simulink library "SKYWARD_LIB_2020b"  (R2020b)
settings: Solver=VariableStepAuto  StartTime=0.0  StopTime=10.0  RelTol=1e-3
undefined symbols (not defined in the file): A_d, CD, h0, I, m, q0, rho
libraries: $bdroot x2
settings Model: Creator=alem1  LastModifiedBy=aless

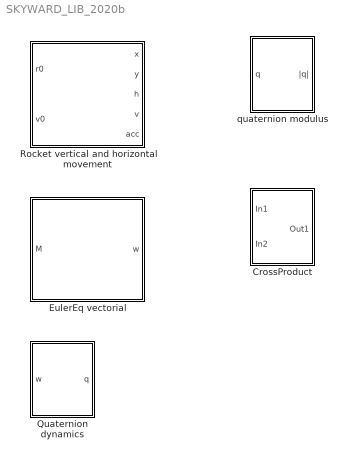
== system SKYWARD_LIB_2020b ==
  CrossProduct : Subsystem
  EulerEq vectorial : Subsystem
  Quaternion dynamics : Subsystem
  Rocket vertical and horizontal movement : Subsystem
  quaternion modulus : Subsystem

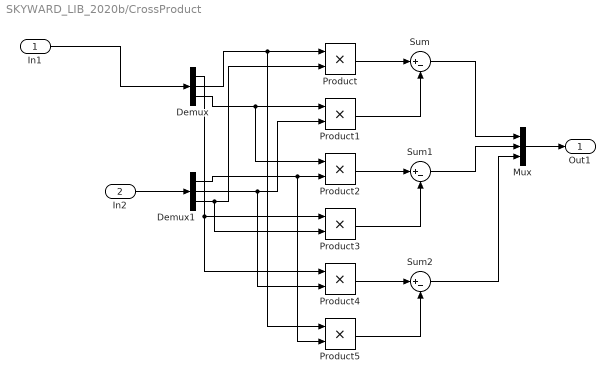
== system SKYWARD_LIB_2020b/CrossProduct ==
  In1 : Inport
  In2 : Inport  Port=2
  Demux : Demux  Outputs=3
  Demux1 : Demux  Outputs=3
  Mux : Mux  Inputs=3
  Product{,1..5} (6 alike) : Product
  Sum : Sum  Inputs=|+-
  Sum1 : Sum  Inputs=|+-
  Sum2 : Sum  Inputs=|+-
  Out1 : Outport
  wires:
  In1/1 -> Demux/1
  Demux1/1 -> Product5/2, Product2/2
  Product/1 -> Sum/1
  Product1/1 -> Sum/2
  Demux1/2 -> Product4/2, Product1/2
  Demux/1 -> Product4/1, Product3/1
  Demux1/3 -> Product3/2, Product/2
  Product3/1 -> Sum1/2
  Sum/1 -> Mux/1
  Product2/1 -> Sum1/1
  Sum1/1 -> Mux/2
  Product4/1 -> Sum2/1
  Product5/1 -> Sum2/2
  Mux/1 -> Out1/1
  Sum2/1 -> Mux/3
  Demux/2 -> Product5/1, Product/1
  In2/1 -> Demux1/1
  Demux/3 -> Product2/1, Product1/1

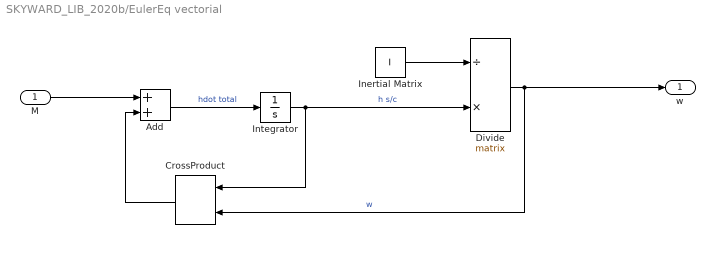
== system SKYWARD_LIB_2020b/EulerEq vectorial ==
  M : Inport
  Add : Sum
  CrossProduct : $bdroot/CrossProduct  SystemSampleTime=-1  VariantActivationTime=update diagram  Latency=0  AutoFrameSizeCalculation=off
  Divide : Product  Inputs=/*  Multiplication=Matrix(*)
  Inertial Matrix : Constant  Value=I
  Integrator : Integrator  InitialCondition=h0
  w : Outport
  wires:
  Integrator/1 -> CrossProduct/1, Divide/2  "h s/c"
  Inertial Matrix/1 -> Divide/1
  Divide/1 -> CrossProduct/2, w/1  "w"
  Add/1 -> Integrator/1  "hdot total"
  CrossProduct/1 -> Add/2
  M/1 -> Add/1

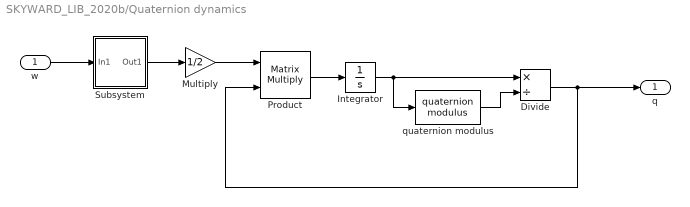
== system SKYWARD_LIB_2020b/Quaternion dynamics ==
  w : Inport
  Divide : Product  Inputs=*/
  Integrator : Integrator  InitialCondition=q0
  Multiply : Gain  Gain=1/2
  Product : Product  Multiplication=Matrix(*)
  Subsystem : Subsystem
  quaternion modulus : $bdroot/quaternion modulus  SystemSampleTime=-1  VariantActivationTime=update diagram  Latency=0  AutoFrameSizeCalculation=off
  q : Outport
  wires:
  Divide/1 -> Product/2, q/1
  quaternion modulus/1 -> Divide/2
  Integrator/1 -> quaternion modulus/1, Divide/1
  Product/1 -> Integrator/1
  Multiply/1 -> Product/1
  Subsystem/1(Out1) -> Multiply/1
  w/1 -> Subsystem/1(In1)

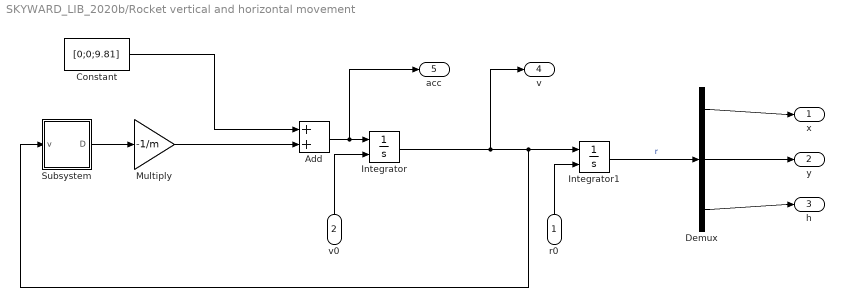
== system SKYWARD_LIB_2020b/Rocket vertical and horizontal movement ==
  r0 : Inport
  v0 : Inport  Port=2
  Add : Sum
  Constant : Constant  Value=[0;0;9.81]
  Demux : Demux  Outputs=3
  Integrator : Integrator  InitialConditionSource=external
  Integrator1 : Integrator  InitialConditionSource=external
  Multiply : Gain  Gain=-1/m
  Subsystem : Subsystem
  x : Outport
  y : Outport  Port=2
  h : Outport  Port=3
  v : Outport  Port=4
  acc : Outport  Port=5
  wires:
  Add/1 -> acc/1, Integrator/1
  v0/1 -> Integrator/2
  Subsystem/1(D) -> Multiply/1
  Demux/1 -> x/1
  Constant/1 -> Add/1
  Multiply/1 -> Add/2
  Integrator1/1 -> Demux/1  "r"
  Integrator/1 -> Subsystem/1(v), Integrator1/1, v/1
  r0/1 -> Integrator1/2
  Demux/2 -> y/1
  Demux/3 -> h/1

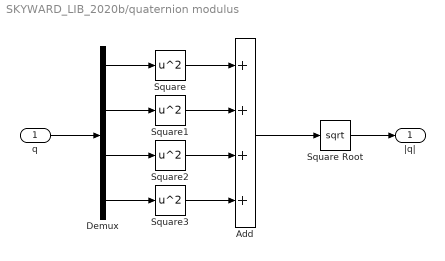
== system SKYWARD_LIB_2020b/quaternion modulus ==
  q : Inport
  Add : Sum  Inputs=++++
  Demux : Demux
  Square{,1..3} (4 alike) : Math  Operator=square  SaturateOnIntegerOverflow=on
  Square Root : Sqrt  SaturateOnIntegerOverflow=on
  |q| : Outport
  wires:
  Square/1 -> Add/1
  Demux/4 -> Square3/1
  q/1 -> Demux/1
  Square3/1 -> Add/4
  Demux/3 -> Square2/1
  Add/1 -> Square Root/1
  Demux/1 -> Square/1
  Demux/2 -> Square1/1
  Square1/1 -> Add/2
  Square2/1 -> Add/3
  Square Root/1 -> |q|/1

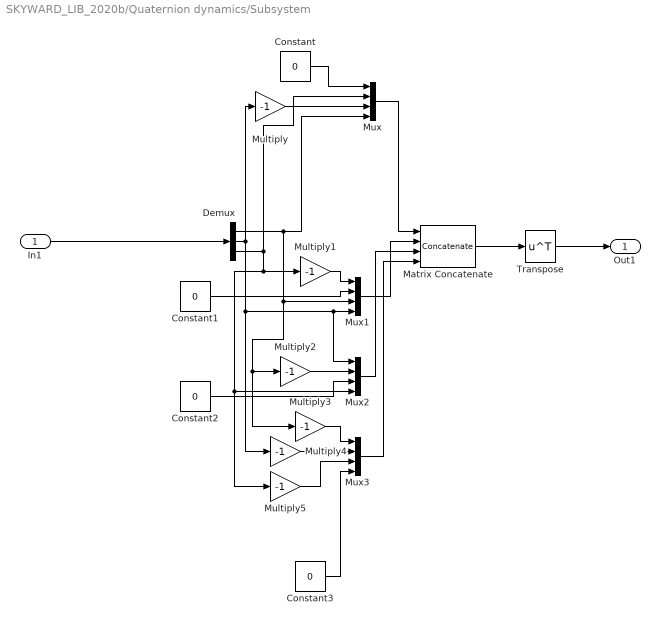
== system SKYWARD_LIB_2020b/Quaternion dynamics/Subsystem ==
  In1 : Inport
  Constant{,1..3} (4 alike) : Constant  Value=0
  Demux : Demux  Outputs=3
  Matrix Concatenate : Concatenate  NumInputs=4  Mode=Multidimensional array  ConcatenateDimension=2
  Multiply{,1..5} (6 alike) : Gain  Gain=-1
  Mux{,1..3} (4 alike) : Mux
  Transpose : Math  Operator=transpose  SaturateOnIntegerOverflow=on
  Out1 : Outport
  wires:
  Transpose/1 -> Out1/1
  Matrix Concatenate/1 -> Transpose/1
  Constant3/1 -> Mux3/4
  Mux2/1 -> Matrix Concatenate/3
  Constant/1 -> Mux/1
  Constant1/1 -> Mux1/2
  Mux/1 -> Matrix Concatenate/1
  Mux1/1 -> Matrix Concatenate/2
  Multiply/1 -> Mux/3
  Mux3/1 -> Matrix Concatenate/4
  Multiply2/1 -> Mux2/2
  Multiply3/1 -> Mux3/1
  Multiply5/1 -> Mux3/3
  Demux/1 -> Multiply3/1, Multiply2/1, Mux1/3, Mux/4
  Demux/3 -> Multiply1/1, Multiply5/1, Mux2/4, Mux/2
  Multiply1/1 -> Mux1/1
  Multiply4/1 -> Mux3/2
  Constant2/1 -> Mux2/3
  In1/1 -> Demux/1
  Demux/2 -> Multiply4/1, Mux2/1, Mux1/4, Multiply/1

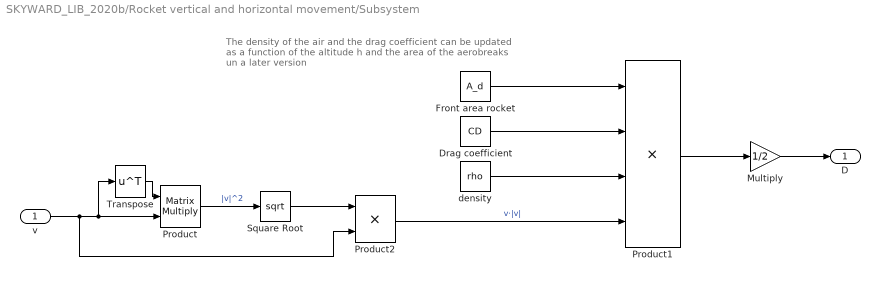
== system SKYWARD_LIB_2020b/Rocket vertical and horizontal movement/Subsystem ==
  note: The density of the air and the drag coefficient can be updated as a function of the altitude h and the area of the aerobreaks un a later version
  v : Inport
  Drag coefficient : Constant  Value=CD
  Front area rocket : Constant  Value=A_d
  Multiply : Gain  Gain=1/2
  Product : Product  Multiplication=Matrix(*)
  Product1 : Product  Inputs=4
  Product2 : Product  Inputs=**
  Square Root : Sqrt  SaturateOnIntegerOverflow=on
  Transpose : Math  Operator=transpose  SaturateOnIntegerOverflow=on
  density : Constant  Value=rho
  D : Outport
  wires:
  Product2/1 -> Product1/4  "v·|v|"
  Product/1 -> Square Root/1  "|v|^2"
  density/1 -> Product1/3
  Square Root/1 -> Product2/1
  Product1/1 -> Multiply/1
  v/1 -> Transpose/1, Product/2, Product2/2
  Multiply/1 -> D/1
  Transpose/1 -> Product/1
  Front area rocket/1 -> Product1/1
  Drag coefficient/1 -> Product1/2
